simulink model "MainPlanevsRainCameras"  (R2020a)
settings: Solver=FixedStepDiscrete  StartTime=0.0  StopTime=20  RelTol=1e-3
model workspace (MAT data in the model file):
  firstWarning = 0
  originalScenarioChecksum = '4AECC2AEC181DD8EA774641D9E64C004'
undefined symbols (not defined in the file): driving
libraries: drivingscenarioandsensors x28
(part 6 of 6)

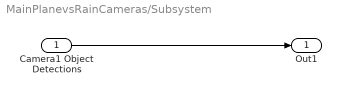
== system MainPlanevsRainCameras/Subsystem ==
  Camera1 Object Detections : Inport
  Out1 : Outport
  wires:
  Camera1 Object Detections/1 -> Out1/1

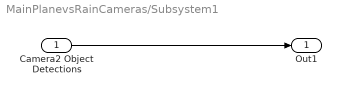
== system MainPlanevsRainCameras/Subsystem1 ==
  Camera2 Object Detections : Inport
  Out1 : Outport
  wires:
  Camera2 Object Detections/1 -> Out1/1

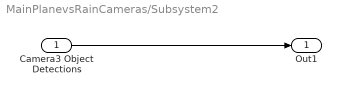
== system MainPlanevsRainCameras/Subsystem2 ==
  Camera3 Object Detections : Inport
  Out1 : Outport
  wires:
  Camera3 Object Detections/1 -> Out1/1

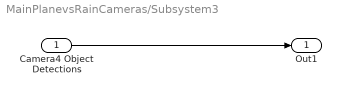
== system MainPlanevsRainCameras/Subsystem3 ==
  Camera4 Object Detections : Inport
  Out1 : Outport
  wires:
  Camera4 Object Detections/1 -> Out1/1

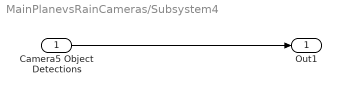
== system MainPlanevsRainCameras/Subsystem4 ==
  Camera5 Object Detections : Inport
  Out1 : Outport
  wires:
  Camera5 Object Detections/1 -> Out1/1

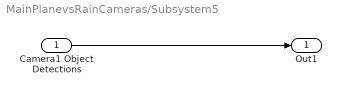
== system MainPlanevsRainCameras/Subsystem5 ==
  Camera1 Object Detections : Inport
  Out1 : Outport
  wires:
  Camera1 Object Detections/1 -> Out1/1

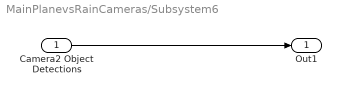
== system MainPlanevsRainCameras/Subsystem6 ==
  Camera2 Object Detections : Inport
  Out1 : Outport
  wires:
  Camera2 Object Detections/1 -> Out1/1

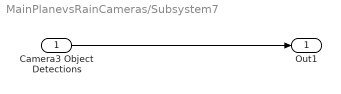
== system MainPlanevsRainCameras/Subsystem7 ==
  Camera3 Object Detections : Inport
  Out1 : Outport
  wires:
  Camera3 Object Detections/1 -> Out1/1

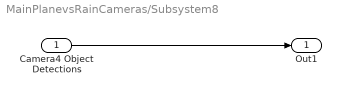
== system MainPlanevsRainCameras/Subsystem8 ==
  Camera4 Object Detections : Inport
  Out1 : Outport
  wires:
  Camera4 Object Detections/1 -> Out1/1

== system MainPlanevsRainCameras/Subsystem9 ==
  Camera5 Object Detections : Inport
  Out1 : Outport
  wires:
  Camera5 Object Detections/1 -> Out1/1
